simulink model "fboard_xaui"  (Simulink 6.2)
settings: Solver=FixedStepDiscrete  SolverMode=SingleTasking  StartTime=0.0  StopTime=10.0  FixedStep=1  RelTol=1e-3
libraries: xbsIndex_r3 x338, fb_xaui x1, newfft_library x1
(part 1 of 3)
settings Model: LastModifiedBy=mdexter
settings DebuggingCC: SolverPrmCheckMsg=warning

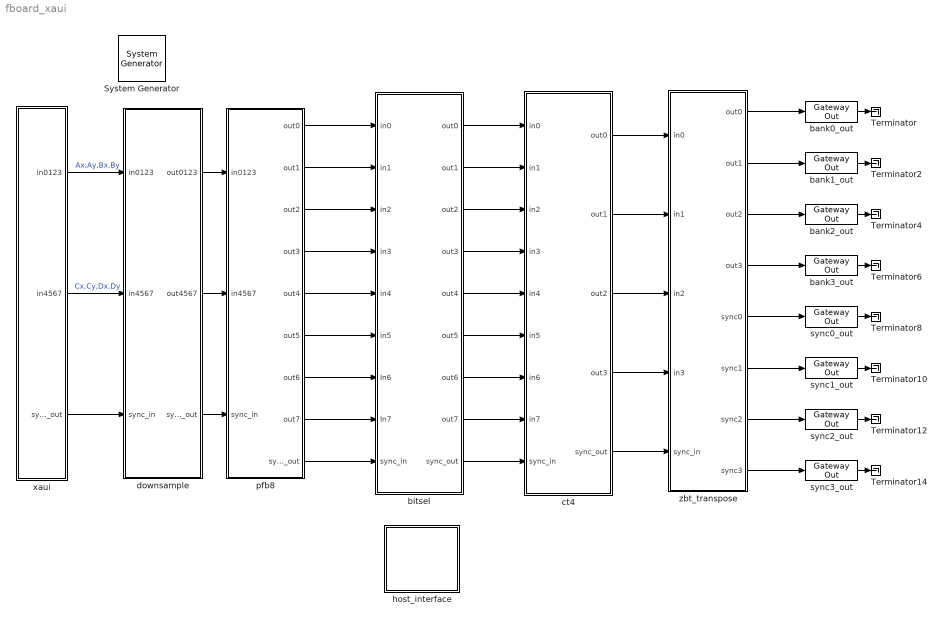
== system fboard_xaui ==
  " System Generator" : xbsIndex_r3/ System Generator  Tag=genX  xilinxfamily=Virtex2P  part=xc2vp40  speed=-6  package=ff1152  synthesis_tool=XST  directory=./netlist  testbench=off  simulink_period=1  sysclk_period=100  incr_netlist=off  trim_vbits=Everywhere in SubSystem  dbl_ovrd=According to Block Masks  core_generation=According to Block Masks  run_coregen=off  deprecated_control=off  eval_field=0
      settings: AttributesFormatString=System\nGenerator
  Terminator{,2,4,6,8,10,12,14} (8 alike) : Terminator
  bank0_out : xbsIndex_r3/Gateway Out  output_type=Double  nbits=8  bin_pt=6  arith_type=Boolean  quantization=Truncate  overflow=Wrap  hdl_port=on  timing_constraint=None  locs_specified=off  LOCs={}  needs_fixed_name=off  show_param=off
      settings: xl_area=[0, 0, 0, 0, 0, 0, 0]
  bank1_out : xbsIndex_r3/Gateway Out  output_type=Double  nbits=8  bin_pt=6  arith_type=Boolean  quantization=Truncate  overflow=Wrap  hdl_port=on  timing_constraint=None  locs_specified=off  LOCs={}  needs_fixed_name=off  show_param=off
      settings: xl_area=[0, 0, 0, 0, 0, 0, 0]
  bank2_out : xbsIndex_r3/Gateway Out  output_type=Double  nbits=8  bin_pt=6  arith_type=Boolean  quantization=Truncate  overflow=Wrap  hdl_port=on  timing_constraint=None  locs_specified=off  LOCs={}  needs_fixed_name=off  show_param=off
      settings: xl_area=[0, 0, 0, 0, 0, 0, 0]
  bank3_out : xbsIndex_r3/Gateway Out  output_type=Double  nbits=8  bin_pt=6  arith_type=Boolean  quantization=Truncate  overflow=Wrap  hdl_port=on  timing_constraint=None  locs_specified=off  LOCs={}  needs_fixed_name=off  show_param=off
      settings: xl_area=[0, 0, 0, 0, 0, 0, 0]
  bitsel : Subsystem
  ct4 : Subsystem
  downsample : Subsystem
  host_interface : Subsystem
  pfb8 : Subsystem
  sync0_out : xbsIndex_r3/Gateway Out  output_type=Double  nbits=8  bin_pt=6  arith_type=Boolean  quantization=Truncate  overflow=Wrap  hdl_port=on  timing_constraint=None  locs_specified=off  LOCs={}  needs_fixed_name=off  show_param=off
      settings: xl_area=[0, 0, 0, 0, 0, 0, 0]
  sync1_out : xbsIndex_r3/Gateway Out  output_type=Double  nbits=8  bin_pt=6  arith_type=Boolean  quantization=Truncate  overflow=Wrap  hdl_port=on  timing_constraint=None  locs_specified=off  LOCs={}  needs_fixed_name=off  show_param=off
      settings: xl_area=[0, 0, 0, 0, 0, 0, 0]
  sync2_out : xbsIndex_r3/Gateway Out  output_type=Double  nbits=8  bin_pt=6  arith_type=Boolean  quantization=Truncate  overflow=Wrap  hdl_port=on  timing_constraint=None  locs_specified=off  LOCs={}  needs_fixed_name=off  show_param=off
      settings: xl_area=[0, 0, 0, 0, 0, 0, 0]
  sync3_out : xbsIndex_r3/Gateway Out  output_type=Double  nbits=8  bin_pt=6  arith_type=Boolean  quantization=Truncate  overflow=Wrap  hdl_port=on  timing_constraint=None  locs_specified=off  LOCs={}  needs_fixed_name=off  show_param=off
      settings: xl_area=[0, 0, 0, 0, 0, 0, 0]
  xaui : Subsystem
  zbt_transpose : Subsystem
  wires:
  pfb8/1(out0) -> bitsel/1(in0)
  pfb8/2(out1) -> bitsel/2(in1)
  pfb8/3(out2) -> bitsel/3(in2)
  pfb8/4(out3) -> bitsel/4(in3)
  pfb8/5(out4) -> bitsel/5(in4)
  pfb8/6(out5) -> bitsel/6(in5)
  pfb8/7(out6) -> bitsel/7(In6)
  pfb8/8(out7) -> bitsel/8(In7)
  pfb8/9(sync_out) -> bitsel/9(sync_in)
  bitsel/1(out0) -> ct4/1(in0)
  ct4/1(out0) -> zbt_transpose/1("in0\t")
  ct4/2(out1) -> zbt_transpose/2(in1)
  ct4/3(out2) -> zbt_transpose/3(in2)
  ct4/4(out3) -> zbt_transpose/4(in3)
  ct4/5(sync_out) -> zbt_transpose/5(sync_in)
  zbt_transpose/1(out0) -> bank0_out/1
  zbt_transpose/2(out1) -> bank1_out/1
  zbt_transpose/3(out2) -> bank2_out/1
  zbt_transpose/4(out3) -> bank3_out/1
  zbt_transpose/5(sync0) -> sync0_out/1
  zbt_transpose/6(sync1) -> sync1_out/1
  zbt_transpose/7(sync2) -> sync2_out/1
  zbt_transpose/8(sync3) -> sync3_out/1
  bitsel/2(out1) -> ct4/2(in1)
  bitsel/3(out2) -> ct4/3(in2)
  bitsel/4(out3) -> ct4/4(in3)
  bitsel/5(out4) -> ct4/5(in4)
  bitsel/6(out5) -> ct4/6(in5)
  bitsel/7(out6) -> ct4/7(in6)
  bitsel/8(out7) -> ct4/8(in7)
  bitsel/9(sync_out) -> ct4/9(sync_in)
  bank0_out/1 -> Terminator/1
  bank1_out/1 -> Terminator2/1
  bank2_out/1 -> Terminator4/1
  bank3_out/1 -> Terminator6/1
  sync0_out/1 -> Terminator8/1
  sync1_out/1 -> Terminator10/1
  sync2_out/1 -> Terminator12/1
  sync3_out/1 -> Terminator14/1
  xaui/1(in0123) -> downsample/1(in0123)  "Ax,Ay,Bx,By"
  xaui/2(in4567) -> downsample/2(in4567)  "Cx,Cy,Dx,Dy"
  xaui/3(sync_out) -> downsample/3(sync_in)
  downsample/1(out0123) -> pfb8/1(in0123)
  downsample/2(out4567) -> pfb8/2(in4567)
  downsample/3(sync_out) -> pfb8/3(sync_in)

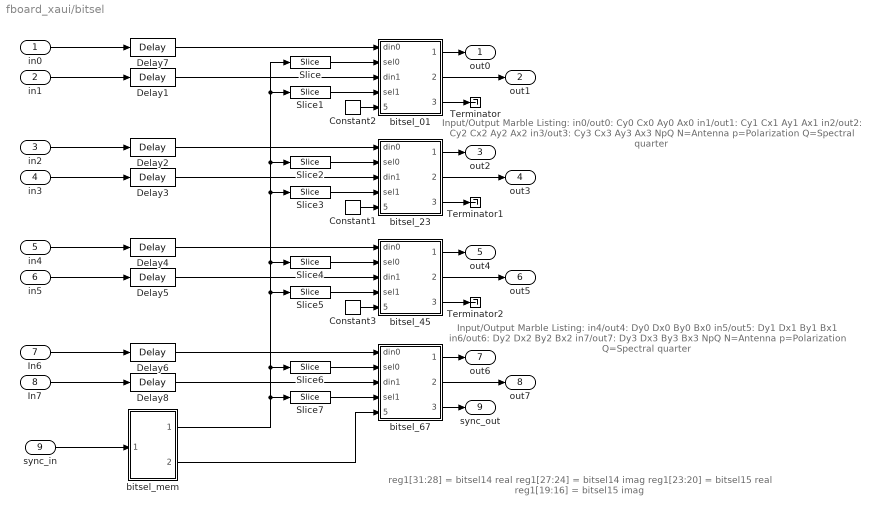
== system fboard_xaui/bitsel ==
  note: Input/Output Marble Listing:
      |
      | in0/out0: Cy0 Cx0 Ay0 Ax0
      | in1/out1: Cy1 Cx1 Ay1 Ax1
      | in2/out2: Cy2 Cx2 Ay2 Ax2
      | in3/out3: Cy3 Cx3 Ay3 Ax3
      |
      | NpQ
      | N=Antenna
      | p=Polarization
      | Q=Spectral quarter
  note: Input/Output Marble Listing:
      |
      | in4/out4: Dy0 Dx0 By0 Bx0
      | in5/out5: Dy1 Dx1 By1 Bx1
      | in6/out6: Dy2 Dx2 By2 Bx2
      | in7/out7: Dy3 Dx3 By3 Bx3
      |
      | NpQ
      | N=Antenna
      | p=Polarization
      | Q=Spectral quarter
  note: reg1[31:28] = bitsel14 real
      | reg1[27:24] = bitsel14 imag
      | reg1[23:20] = bitsel15 real
      | reg1[19:16] = bitsel15 imag
  in0 : Inport  Port=1  LatchInput=off
  in1 : Inport  Port=2  LatchInput=off
  in2 : Inport  Port=3  LatchInput=off
  in3 : Inport  Port=4  LatchInput=off
  in4 : Inport  Port=5  LatchInput=off
  in5 : Inport  Port=6  LatchInput=off
  In6 : Inport  Port=7  LatchInput=off
  In7 : Inport  Port=8  LatchInput=off
  sync_in : Inport  Port=9  LatchInput=off
  Constant1 : xbsIndex_r3/Constant  const=0  equ=P=C  arith_type=Boolean  n_bits=1  bin_pt=0  opselect=C  inp2=PCIN>>17  opr=+  inp1=P  carry=CIN  iostate=0  explicit_period=on  period=1  dbl_ovrd=off
  Constant2 : xbsIndex_r3/Constant  const=0  equ=P=C  arith_type=Boolean  n_bits=1  bin_pt=0  opselect=C  inp2=PCIN>>17  opr=+  inp1=P  carry=CIN  iostate=0  explicit_period=on  period=1  dbl_ovrd=off
  Constant3 : xbsIndex_r3/Constant  const=0  equ=P=C  arith_type=Boolean  n_bits=1  bin_pt=0  opselect=C  inp2=PCIN>>17  opr=+  inp1=P  carry=CIN  iostate=0  explicit_period=on  period=1  dbl_ovrd=off
  Delay{1..8} (8 alike) : xbsIndex_r3/Delay  latency=4  reg_retiming=off  explicit_period=off  period=1  en=off  accept_only_valid=off  init_zero=on  dbl_ovrd=off  show_param=off
      settings: xl_area=[0, 0, 0, 0, 0, 0, 0]
  Slice : xbsIndex_r3/Slice  mode=Lower Bit Location + Width  nbits=4  bit1=0  base1=MSB of Input  bit0=0  base0=LSB of Input  boolean_output=off  explicit_period=off  period=1  dbl_ovrd=off
  Slice1 : xbsIndex_r3/Slice  mode=Lower Bit Location + Width  nbits=4  bit1=0  base1=MSB of Input  bit0=4  base0=LSB of Input  boolean_output=off  explicit_period=off  period=1  dbl_ovrd=off
  Slice2 : xbsIndex_r3/Slice  mode=Lower Bit Location + Width  nbits=4  bit1=0  base1=MSB of Input  bit0=8  base0=LSB of Input  boolean_output=off  explicit_period=off  period=1  dbl_ovrd=off
  Slice3 : xbsIndex_r3/Slice  mode=Lower Bit Location + Width  nbits=4  bit1=0  base1=MSB of Input  bit0=12  base0=LSB of Input  boolean_output=off  explicit_period=off  period=1  dbl_ovrd=off
  Slice4 : xbsIndex_r3/Slice  mode=Lower Bit Location + Width  nbits=4  bit1=0  base1=MSB of Input  bit0=16  base0=LSB of Input  boolean_output=off  explicit_period=off  period=1  dbl_ovrd=off
  Slice5 : xbsIndex_r3/Slice  mode=Lower Bit Location + Width  nbits=4  bit1=0  base1=MSB of Input  bit0=20  base0=LSB of Input  boolean_output=off  explicit_period=off  period=1  dbl_ovrd=off
  Slice6 : xbsIndex_r3/Slice  mode=Lower Bit Location + Width  nbits=4  bit1=0  base1=MSB of Input  bit0=24  base0=LSB of Input  boolean_output=off  explicit_period=off  period=1  dbl_ovrd=off
  Slice7 : xbsIndex_r3/Slice  mode=Lower Bit Location + Width  nbits=4  bit1=0  base1=MSB of Input  bit0=28  base0=LSB of Input  boolean_output=off  explicit_period=off  period=1  dbl_ovrd=off
  Terminator : Terminator
  Terminator1 : Terminator
  Terminator2 : Terminator
  bitsel_01 : Subsystem
  bitsel_23 : Subsystem
  bitsel_45 : Subsystem
  bitsel_67 : Subsystem
  bitsel_mem : Subsystem
      settings: AttributesFormatString=Latency=4
  out0 : Outport
  out1 : Outport  Port=2
  out2 : Outport  Port=3
  out3 : Outport  Port=4
  out4 : Outport  Port=5
  out5 : Outport  Port=6
  out6 : Outport  Port=7
  out7 : Outport  Port=8
  sync_out : Outport  Port=9
  wires:
  in0/1 -> Delay7/1
  bitsel_01/1(dout0) -> out0/1
  in1/1 -> Delay1/1
  in2/1 -> Delay2/1
  in3/1 -> Delay3/1
  in4/1 -> Delay4/1
  in5/1 -> Delay5/1
  In6/1 -> Delay6/1
  In7/1 -> Delay8/1
  bitsel_mem/2(sync_out) -> bitsel_67/5(sync_in)
  Slice/1 -> bitsel_01/2(sel0)
  Slice1/1 -> bitsel_01/4(sel1)
  Slice2/1 -> bitsel_23/2(sel0)
  Slice3/1 -> bitsel_23/4(sel1)
  Slice4/1 -> bitsel_45/2(sel0)
  Slice5/1 -> bitsel_45/4(sel1)
  Slice6/1 -> bitsel_67/2(sel0)
  Slice7/1 -> bitsel_67/4(sel1)
  bitsel_mem/1(bitsel) -> Slice5/1, Slice4/1, Slice3/1, Slice2/1, Slice/1, Slice1/1, Slice6/1, Slice7/1
  bitsel_01/3(sync_out) -> Terminator/1
  bitsel_01/2(dout1) -> out1/1
  bitsel_23/1(dout0) -> out2/1
  bitsel_23/3(sync_out) -> Terminator1/1
  bitsel_23/2(dout1) -> out3/1
  bitsel_45/1(dout0) -> out4/1
  bitsel_45/3(sync_out) -> Terminator2/1
  bitsel_45/2(dout1) -> out5/1
  bitsel_67/1(dout0) -> out6/1
  bitsel_67/2(dout1) -> out7/1
  bitsel_67/3(sync_out) -> sync_out/1
  sync_in/1 -> bitsel_mem/1(sync_in)
  Constant2/1 -> bitsel_01/5(sync_in)
  Constant3/1 -> bitsel_45/5(sync_in)
  Constant1/1 -> bitsel_23/5(sync_in)
  Delay7/1 -> bitsel_01/1(din0)
  Delay1/1 -> bitsel_01/3(din1)
  Delay2/1 -> bitsel_23/1(din0)
  Delay3/1 -> bitsel_23/3(din1)
  Delay4/1 -> bitsel_45/1(din0)
  Delay5/1 -> bitsel_45/3(din1)
  Delay6/1 -> bitsel_67/1(din0)
  Delay8/1 -> bitsel_67/3(din1)

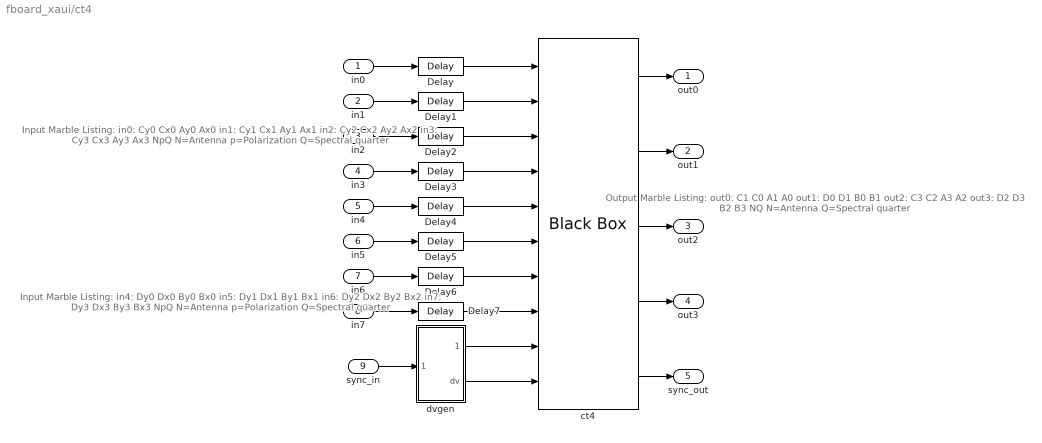
== system fboard_xaui/ct4 ==
  note: Input Marble Listing:
      |
      | in0: Cy0 Cx0 Ay0 Ax0
      | in1: Cy1 Cx1 Ay1 Ax1
      | in2: Cy2 Cx2 Ay2 Ax2
      | in3: Cy3 Cx3 Ay3 Ax3
      |
      | NpQ
      | N=Antenna
      | p=Polarization
      | Q=Spectral quarter
  note: Input Marble Listing:
      |
      | in4: Dy0 Dx0 By0 Bx0
      | in5: Dy1 Dx1 By1 Bx1
      | in6: Dy2 Dx2 By2 Bx2
      | in7: Dy3 Dx3 By3 Bx3
      |
      | NpQ
      | N=Antenna
      | p=Polarization
      | Q=Spectral quarter
  note: Output Marble Listing:
      |
      | out0: C1 C0 A1 A0
      | out1: D0 D1 B0 B1
      | out2: C3 C2 A3 A2
      | out3: D2 D3 B2 B3
      |
      | NQ
      | N=Antenna
      | Q=Spectral quarter
  in0 : Inport  Port=1  LatchInput=off
  in1 : Inport  Port=2  LatchInput=off
  in2 : Inport  Port=3  LatchInput=off
  in3 : Inport  Port=4  LatchInput=off
  in4 : Inport  Port=5  LatchInput=off
  in5 : Inport  Port=6  LatchInput=off
  in6 : Inport  Port=7  LatchInput=off
  in7 : Inport  Port=8  LatchInput=off
  sync_in : Inport  Port=9  LatchInput=off
  Delay{,1..7} (8 alike) : xbsIndex_r3/Delay  latency=3  reg_retiming=off  explicit_period=off  period=1  en=off  accept_only_valid=off  init_zero=on  dbl_ovrd=off  show_param=off
      settings: xl_area=[0, 0, 0, 0, 0, 0, 0]
  ct4 : xbsIndex_r3/Black Box  init_code=ct4_dv_config  sim_method=Inactive  show_param=off
      settings: xl_area=[0, 0, 0, 0, 0, 0, 0]
  dvgen : Subsystem
      settings: AttributesFormatString=Latency=3
  out0 : Outport
  out1 : Outport  Port=2
  out2 : Outport  Port=3
  out3 : Outport  Port=4
  sync_out : Outport  Port=5
  wires:
  in0/1 -> Delay/1
  ct4/1 -> out0/1
  in1/1 -> Delay1/1
  ct4/2 -> out1/1
  in2/1 -> Delay2/1
  ct4/3 -> out2/1
  in3/1 -> Delay3/1
  ct4/4 -> out3/1
  in4/1 -> Delay4/1
  ct4/5 -> sync_out/1
  in5/1 -> Delay5/1
  in6/1 -> Delay6/1
  in7/1 -> Delay7/1
  dvgen/1(sync_out) -> ct4/9
  dvgen/2(dv) -> ct4/10
  sync_in/1 -> dvgen/1(sync_in)
  Delay/1 -> ct4/1
  Delay1/1 -> ct4/2
  Delay2/1 -> ct4/3
  Delay3/1 -> ct4/4
  Delay4/1 -> ct4/5
  Delay5/1 -> ct4/6
  Delay6/1 -> ct4/7
  Delay7/1 -> ct4/8

== system fboard_xaui/downsample ==
  note: The down-sampling step down-samples the sync pulse to the
      | slower rate and down-samples data to the slower rate as well.
  note: sync_in (1/1 rate): _S_____________
      | data_in (1/1 rate): YZ0123456789ABC
      | sync_out (1/2 rate): _____SS________
      | data_out (1/2 rate): TVVXXZZ11335577
      | dv (1/2 rate): 010101010101010
  in0123 : Inport  Port=1  LatchInput=off
  in4567 : Inport  Port=2  LatchInput=off
  sync_in : Inport  Port=3  LatchInput=off
  Delay1 : xbsIndex_r3/Delay  latency=3  reg_retiming=off  explicit_period=off  period=1  en=off  accept_only_valid=off  init_zero=on  dbl_ovrd=off  show_param=off
      settings: xl_area=[0, 0, 0, 0, 0, 0, 0]
  Delay2 : xbsIndex_r3/Delay  latency=3  reg_retiming=off  explicit_period=off  period=1  en=off  accept_only_valid=off  init_zero=on  dbl_ovrd=off  show_param=off
      settings: xl_area=[0, 0, 0, 0, 0, 0, 0]
  Register : xbsIndex_r3/Register  init=0  reg_only_valid=off  explicit_period=off  period=1  rst=off  en=on  out_en=off  dbl_ovrd=off  show_param=off
      settings: xl_area=[0, 0, 0, 0, 0, 0, 0]
  Register1 : xbsIndex_r3/Register  init=0  reg_only_valid=off  explicit_period=off  period=1  rst=off  en=on  out_en=off  dbl_ovrd=off  show_param=off
      settings: xl_area=[0, 0, 0, 0, 0, 0, 0]
  Register2 : xbsIndex_r3/Register  init=0  reg_only_valid=off  explicit_period=off  period=1  rst=off  en=on  out_en=off  dbl_ovrd=off  show_param=off
      settings: xl_area=[0, 0, 0, 0, 0, 0, 0]
  dvgen : Subsystem
      settings: AttributesFormatString=Latency=3
  out0123 : Outport
  out4567 : Outport  Port=2
  sync_out : Outport  Port=3
  wires:
  in0123/1 -> Delay1/1
  in4567/1 -> Delay2/1
  sync_in/1 -> dvgen/1(sync_in)
  Register/1 -> out0123/1
  Register1/1 -> out4567/1
  Register2/1 -> sync_out/1
  dvgen/1(sync_out) -> Register2/1
  dvgen/2(dv) -> Register2/2, Register/2, Register1/2
  Delay1/1 -> Register/1
  Delay2/1 -> Register1/1

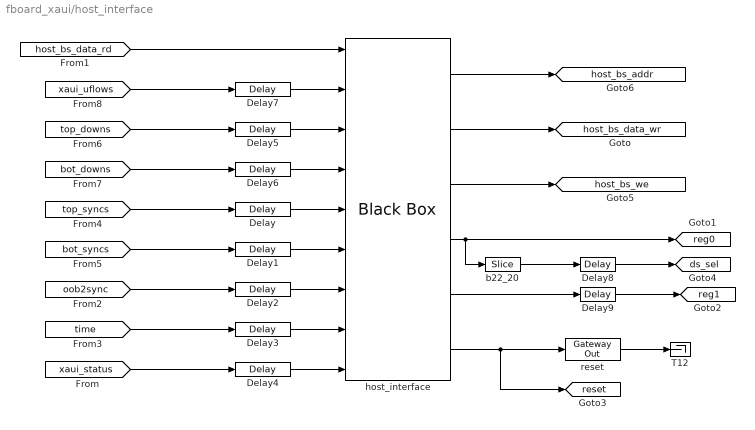
== system fboard_xaui/host_interface ==
  Delay{,1..7} (8 alike) : xbsIndex_r3/Delay  latency=1  reg_retiming=off  explicit_period=off  period=1  en=off  accept_only_valid=off  init_zero=on  dbl_ovrd=off  show_param=off
      settings: xl_area=[0, 0, 0, 0, 0, 0, 0]
  Delay8 : xbsIndex_r3/Delay  latency=3  reg_retiming=on  explicit_period=off  period=1  en=off  accept_only_valid=off  init_zero=on  dbl_ovrd=off  show_param=off
      settings: xl_area=[0, 0, 0, 0, 0, 0, 0]
  Delay9 : xbsIndex_r3/Delay  latency=3  reg_retiming=on  explicit_period=off  period=1  en=off  accept_only_valid=off  init_zero=on  dbl_ovrd=off  show_param=off
      settings: xl_area=[0, 0, 0, 0, 0, 0, 0]
  T12 : Terminator
  b22_20 : xbsIndex_r3/Slice  mode=Lower Bit Location + Width  nbits=3  bit1=0  base1=MSB of Input  bit0=20  base0=LSB of Input  boolean_output=off  explicit_period=off  period=1  dbl_ovrd=off
  host_interface : xbsIndex_r3/Black Box  init_code=host_interface_config  sim_method=Inactive  show_param=off
      settings: xl_area=[0, 0, 0, 0, 0, 0, 0]
  reset : xbsIndex_r3/Gateway Out  output_type=Double  nbits=8  bin_pt=6  arith_type=Boolean  quantization=Truncate  overflow=Wrap  hdl_port=on  timing_constraint=None  locs_specified=off  LOCs={}  needs_fixed_name=off  show_param=off
      settings: xl_area=[0, 0, 0, 0, 0, 0, 0]
  tag scope: ds_sel=global, host_bs_addr=global, host_bs_data_wr=global, host_bs_we=global, reg0=global, reg1=global, reset=global
  wires:
  reset/1 -> T12/1
  [host_bs_data_rd] -> host_interface/1
  host_interface/6 -> reset/1, [reset]
  host_interface/2 -> [host_bs_data_wr]
  [top_syncs] -> Delay/1
  [bot_syncs] -> Delay1/1
  [oob2sync] -> Delay2/1
  [time] -> Delay3/1
  [xaui_status] -> Delay4/1
  [top_downs] -> Delay5/1
  [bot_downs] -> Delay6/1
  host_interface/4 -> [reg0], b22_20/1
  host_interface/5 -> Delay9/1
  [xaui_uflows] -> Delay7/1
  Delay7/1 -> host_interface/2
  Delay5/1 -> host_interface/3
  Delay6/1 -> host_interface/4
  Delay/1 -> host_interface/5
  Delay1/1 -> host_interface/6
  Delay2/1 -> host_interface/7
  Delay3/1 -> host_interface/8
  Delay4/1 -> host_interface/9
  b22_20/1 -> Delay8/1
  host_interface/3 -> [host_bs_we]
  host_interface/1 -> [host_bs_addr]
  Delay8/1 -> [ds_sel]
  Delay9/1 -> [reg1]

== system fboard_xaui/pfb8 ==
  in0123 : Inport  Port=1  LatchInput=off
  in4567 : Inport  Port=2  LatchInput=off
  sync_in : Inport  Port=3  LatchInput=off
  b64x1_b16x4_bot : Subsystem
  b64x1_b16x4_top : Subsystem
  fir8 : Subsystem  mask{fb_ntaps=4}
      mask prompts: fb_ntaps "Number of taps"
  pfb_fft8 : Subsystem
  out0 : Outport
  out1 : Outport  Port=2
  out2 : Outport  Port=3
  out3 : Outport  Port=4
  out4 : Outport  Port=5
  out5 : Outport  Port=6
  out6 : Outport  Port=7
  out7 : Outport  Port=8
  sync_out : Outport  Port=9
  wires:
  fir8/8(out7) -> pfb_fft8/8(in7)
  fir8/7(out6) -> pfb_fft8/7(in6)
  fir8/9(sync_out) -> pfb_fft8/9(sync_in)
  fir8/6(out5) -> pfb_fft8/6(in5)
  fir8/5(out4) -> pfb_fft8/5(in4)
  fir8/4(out3) -> pfb_fft8/4(in3)
  fir8/3(out2) -> pfb_fft8/3(in2)
  fir8/2(out1) -> pfb_fft8/2(in1)
  fir8/1(out0) -> pfb_fft8/1(in0)
  b64x1_b16x4_top/2(dout1) -> fir8/2(in1)
  b64x1_b16x4_top/1(dout0) -> fir8/1(in0)
  b64x1_b16x4_bot/4(dout3) -> fir8/8(in7)
  b64x1_b16x4_bot/3(dout2) -> fir8/7(in6)
  b64x1_b16x4_bot/2(dout1) -> fir8/6(in5)
  b64x1_b16x4_bot/1(dout0) -> fir8/5(in4)
  b64x1_b16x4_top/4(dout3) -> fir8/4(in3)
  b64x1_b16x4_top/3(dout2) -> fir8/3(in2)
  pfb_fft8/1(out0) -> out0/1
  pfb_fft8/2(out1) -> out1/1
  in0123/1 -> b64x1_b16x4_top/1(din)
  pfb_fft8/3(out2) -> out2/1
  pfb_fft8/4(out3) -> out3/1
  pfb_fft8/5(out4) -> out4/1
  pfb_fft8/6(out5) -> out5/1
  in4567/1 -> b64x1_b16x4_bot/1(din)
  pfb_fft8/7(out6) -> out6/1
  pfb_fft8/8(out7) -> out7/1
  pfb_fft8/9(sync_out) -> sync_out/1
  sync_in/1 -> fir8/9(sync_in)

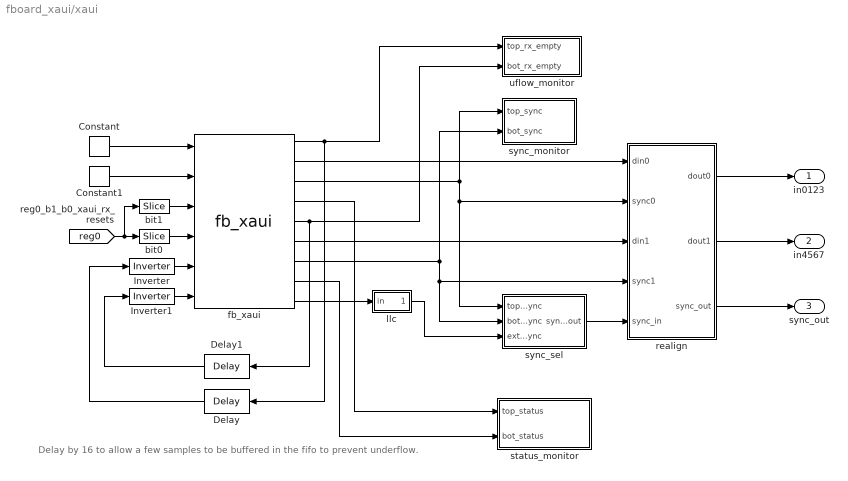
== system fboard_xaui/xaui ==
  note: Delay by 16 to allow a few samples to be
      | buffered in the fifo to prevent underflow.
  Constant : xbsIndex_r3/Constant  const=0  equ=P=C  arith_type=Boolean  n_bits=1  bin_pt=0  opselect=C  inp2=PCIN>>17  opr=+  inp1=P  carry=CIN  iostate=0  explicit_period=on  period=1  dbl_ovrd=off
  Constant1 : xbsIndex_r3/Constant  const=1  equ=P=C  arith_type=Boolean  n_bits=1  bin_pt=0  opselect=C  inp2=PCIN>>17  opr=+  inp1=P  carry=CIN  iostate=0  explicit_period=on  period=1  dbl_ovrd=off
  Delay : xbsIndex_r3/Delay  Orientation=left  latency=16  reg_retiming=off  explicit_period=off  period=1  en=off  accept_only_valid=off  init_zero=on  dbl_ovrd=off  show_param=off
      settings: xl_area=[0, 0, 0, 0, 0, 0, 0]
  Delay1 : xbsIndex_r3/Delay  Orientation=left  latency=16  reg_retiming=off  explicit_period=off  period=1  en=off  accept_only_valid=off  init_zero=on  dbl_ovrd=off  show_param=off
      settings: xl_area=[0, 0, 0, 0, 0, 0, 0]
  Inverter : xbsIndex_r3/Inverter  latency=0  explicit_period=off  period=1  en=off  dbl_ovrd=off  show_param=off
      settings: xl_area=[0, 0, 0, 0, 0, 0, 0]
  Inverter1 : xbsIndex_r3/Inverter  latency=0  explicit_period=off  period=1  en=off  dbl_ovrd=off  show_param=off
      settings: xl_area=[0, 0, 0, 0, 0, 0, 0]
  bit0 : xbsIndex_r3/Slice  mode=Lower Bit Location + Width  nbits=1  bit1=12  base1=MSB of Input  bit0=0  base0=LSB of Input  boolean_output=on  explicit_period=off  period=1  dbl_ovrd=off
  bit1 : xbsIndex_r3/Slice  mode=Lower Bit Location + Width  nbits=1  bit1=12  base1=MSB of Input  bit0=1  base0=LSB of Input  boolean_output=on  explicit_period=off  period=1  dbl_ovrd=off
  fb_xaui : fb_xaui/fb_xaui
  llc : Subsystem
  realign : Subsystem
  status_monitor : Subsystem
  sync_monitor : Subsystem
  sync_sel : Subsystem
  uflow_monitor : Subsystem
  in0123 : Outport
  in4567 : Outport  Port=2
  sync_out : Outport  Port=3
  wires:
  Constant/1 -> fb_xaui/1
  Constant1/1 -> fb_xaui/2
  fb_xaui/8 -> status_monitor/2(bot_status)
  fb_xaui/4 -> status_monitor/1(top_status)
  fb_xaui/2 -> realign/1(din0)
  fb_xaui/3 -> sync_monitor/1(top_sync), sync_sel/1(top_sync), realign/2(sync0)
  fb_xaui/6 -> realign/3(din1)
  fb_xaui/7 -> sync_monitor/2(bot_sync), realign/4(sync1), sync_sel/2(bot_sync)
  realign/1(dout0) -> in0123/1
  realign/2(dout1) -> in4567/1
  realign/3(sync_out) -> sync_out/1
  sync_sel/1(sync_out) -> realign/5(sync_in)
  fb_xaui/1 -> uflow_monitor/1(top_rx_empty), Delay/1
  fb_xaui/5 -> uflow_monitor/2(bot_rx_empty), Delay1/1
  [reg0] -> bit0/1, bit1/1
  bit1/1 -> fb_xaui/3
  bit0/1 -> fb_xaui/4
  Delay/1 -> Inverter/1
  Delay1/1 -> Inverter1/1
  Inverter/1 -> fb_xaui/5
  Inverter1/1 -> fb_xaui/6
  fb_xaui/9 -> llc/1(in)
  llc/1(out) -> sync_sel/3(ext_sync)

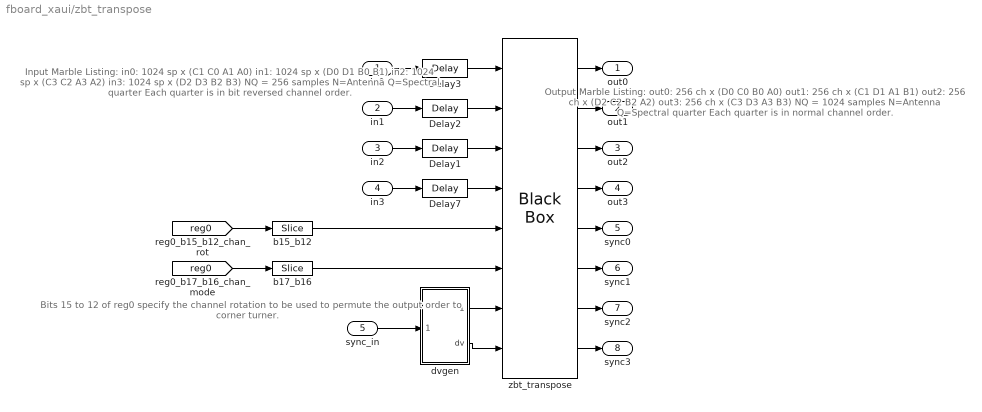
== system fboard_xaui/zbt_transpose ==
  note: Input Marble Listing:
      |
      | in0: 1024 sp x (C1 C0 A1 A0)
      | in1: 1024 sp x (D0 D1 B0 B1)
      | in2: 1024 sp x (C3 C2 A3 A2)
      | in3: 1024 sp x (D2 D3 B2 B3)
      |
      | NQ = 256 samples
      |
      | N=Antenna
      | Q=Spectral quarter
      |
      | Each quarter is in bit
      | reversed channel order.
  note: Output Marble Listing:
      |
      | out0: 256 ch x (D0 C0 B0 A0)
      | out1: 256 ch x (C1 D1 A1 B1)
      | out2: 256 ch x (D2 C2 B2 A2)
      | out3: 256 ch x (C3 D3 A3 B3)
      |
      | NQ = 1024 samples
      |
      | N=Antenna
      | Q=Spectral quarter
      |
      | Each quarter is in
      | normal channel order.
  note: Bits 15 to 12 of reg0
      | specify the channel rotation
      | to be used to permute the
      | output order to corner turner.
  "in0\t" : Inport  Port=1  LatchInput=off
  in1 : Inport  Port=2  LatchInput=off
  in2 : Inport  Port=3  LatchInput=off
  in3 : Inport  Port=4  LatchInput=off
  sync_in : Inport  Port=5  LatchInput=off
  Delay{1..3,7} (4 alike) : xbsIndex_r3/Delay  latency=3  reg_retiming=off  explicit_period=off  period=1  en=off  accept_only_valid=off  init_zero=on  dbl_ovrd=off  show_param=off
      settings: xl_area=[0, 0, 0, 0, 0, 0, 0]
  b15_b12 : xbsIndex_r3/Slice  mode=Lower Bit Location + Width  nbits=4  bit1=12  base1=MSB of Input  bit0=12  base0=LSB of Input  boolean_output=off  explicit_period=off  period=1  dbl_ovrd=off
  b17_b16 : xbsIndex_r3/Slice  mode=Lower Bit Location + Width  nbits=2  bit1=12  base1=MSB of Input  bit0=16  base0=LSB of Input  boolean_output=off  explicit_period=off  period=1  dbl_ovrd=off
  dvgen : Subsystem
      settings: AttributesFormatString=Latency=3
  zbt_transpose : xbsIndex_r3/Black Box  init_code=zbt_transpose_config  sim_method=Inactive  show_param=off
      settings: xl_area=[0, 0, 0, 0, 0, 0, 0]
  out0 : Outport
  out1 : Outport  Port=2
  out2 : Outport  Port=3
  out3 : Outport  Port=4
  sync0 : Outport  Port=5
  sync1 : Outport  Port=6
  sync2 : Outport  Port=7
  sync3 : Outport  Port=8
  wires:
  zbt_transpose/1 -> out0/1
  "in0\t"/1 -> Delay3/1
  zbt_transpose/2 -> out1/1
  in1/1 -> Delay2/1
  zbt_transpose/3 -> out2/1
  zbt_transpose/4 -> out3/1
  in2/1 -> Delay1/1
  zbt_transpose/5 -> sync0/1
  in3/1 -> Delay7/1
  zbt_transpose/6 -> sync1/1
  zbt_transpose/7 -> sync2/1
  zbt_transpose/8 -> sync3/1
  [reg0] -> b15_b12/1
  [reg0] -> b17_b16/1
  b15_b12/1 -> zbt_transpose/5
  b17_b16/1 -> zbt_transpose/6
  Delay7/1 -> zbt_transpose/4
  Delay1/1 -> zbt_transpose/3
  Delay2/1 -> zbt_transpose/2
  Delay3/1 -> zbt_transpose/1
  dvgen/1(sync_out) -> zbt_transpose/7
  dvgen/2(dv) -> zbt_transpose/8
  sync_in/1 -> dvgen/1(sync_in)

== system fboard_xaui/bitsel/bitsel_01 ==
  din0 : Inport  Port=1  LatchInput=off
  sel0 : Inport  Port=2  LatchInput=off
  din1 : Inport  Port=3  LatchInput=off
  sel1 : Inport  Port=4  LatchInput=off
  sync_in : Inport  Port=5  LatchInput=off
  Constant : xbsIndex_r3/Constant  const=0  equ=P=C  arith_type=Boolean  n_bits=1  bin_pt=0  opselect=C  inp2=PCIN>>17  opr=+  inp1=P  carry=CIN  iostate=0  explicit_period=on  period=1  dbl_ovrd=off
  Terminator : Terminator
  bitsel_0 : xbsIndex_r3/Black Box  init_code=bitsel_config  sim_method=Inactive  show_param=off
      settings: xl_area=[0, 0, 0, 0, 0, 0, 0]
  bitsel_1 : xbsIndex_r3/Black Box  init_code=bitsel_config  sim_method=Inactive  show_param=off
      settings: xl_area=[0, 0, 0, 0, 0, 0, 0]
  dout0 : Outport
  dout1 : Outport  Port=2
  sync_out : Outport  Port=3
  wires:
  din0/1 -> bitsel_0/1
  din1/1 -> bitsel_1/1
  sel0/1 -> bitsel_0/2
  bitsel_0/1 -> dout0/1
  sel1/1 -> bitsel_1/2
  bitsel_1/1 -> dout1/1
  sync_in/1 -> bitsel_1/4
  bitsel_1/2 -> sync_out/1
  bitsel_0/2 -> Terminator/1
  Constant/1 -> bitsel_0/4
  [bs1415] -> bitsel_0/3
  [bs1415] -> bitsel_1/3

== system fboard_xaui/bitsel/bitsel_23 ==
  din0 : Inport  Port=1  LatchInput=off
  sel0 : Inport  Port=2  LatchInput=off
  din1 : Inport  Port=3  LatchInput=off
  sel1 : Inport  Port=4  LatchInput=off
  sync_in : Inport  Port=5  LatchInput=off
  Constant : xbsIndex_r3/Constant  const=0  equ=P=C  arith_type=Boolean  n_bits=1  bin_pt=0  opselect=C  inp2=PCIN>>17  opr=+  inp1=P  carry=CIN  iostate=0  explicit_period=on  period=1  dbl_ovrd=off
  Terminator : Terminator
  bitsel_0 : xbsIndex_r3/Black Box  init_code=bitsel_config  sim_method=Inactive  show_param=off
      settings: xl_area=[0, 0, 0, 0, 0, 0, 0]
  bitsel_1 : xbsIndex_r3/Black Box  init_code=bitsel_config  sim_method=Inactive  show_param=off
      settings: xl_area=[0, 0, 0, 0, 0, 0, 0]
  dout0 : Outport
  dout1 : Outport  Port=2
  sync_out : Outport  Port=3
  wires:
  din0/1 -> bitsel_0/1
  din1/1 -> bitsel_1/1
  sel0/1 -> bitsel_0/2
  bitsel_0/1 -> dout0/1
  sel1/1 -> bitsel_1/2
  bitsel_1/1 -> dout1/1
  sync_in/1 -> bitsel_1/4
  bitsel_1/2 -> sync_out/1
  bitsel_0/2 -> Terminator/1
  Constant/1 -> bitsel_0/4
  [bs1415] -> bitsel_0/3
  [bs1415] -> bitsel_1/3

== system fboard_xaui/bitsel/bitsel_45 ==
  din0 : Inport  Port=1  LatchInput=off
  sel0 : Inport  Port=2  LatchInput=off
  din1 : Inport  Port=3  LatchInput=off
  sel1 : Inport  Port=4  LatchInput=off
  sync_in : Inport  Port=5  LatchInput=off
  Constant : xbsIndex_r3/Constant  const=0  equ=P=C  arith_type=Boolean  n_bits=1  bin_pt=0  opselect=C  inp2=PCIN>>17  opr=+  inp1=P  carry=CIN  iostate=0  explicit_period=on  period=1  dbl_ovrd=off
  Terminator : Terminator
  bitsel_0 : xbsIndex_r3/Black Box  init_code=bitsel_config  sim_method=Inactive  show_param=off
      settings: xl_area=[0, 0, 0, 0, 0, 0, 0]
  bitsel_1 : xbsIndex_r3/Black Box  init_code=bitsel_config  sim_method=Inactive  show_param=off
      settings: xl_area=[0, 0, 0, 0, 0, 0, 0]
  dout0 : Outport
  dout1 : Outport  Port=2
  sync_out : Outport  Port=3
  wires:
  din0/1 -> bitsel_0/1
  din1/1 -> bitsel_1/1
  sel0/1 -> bitsel_0/2
  bitsel_0/1 -> dout0/1
  sel1/1 -> bitsel_1/2
  bitsel_1/1 -> dout1/1
  sync_in/1 -> bitsel_1/4
  bitsel_1/2 -> sync_out/1
  bitsel_0/2 -> Terminator/1
  Constant/1 -> bitsel_0/4
  [bs1415] -> bitsel_0/3
  [bs1415] -> bitsel_1/3

== system fboard_xaui/bitsel/bitsel_67 ==
  din0 : Inport  Port=1  LatchInput=off
  sel0 : Inport  Port=2  LatchInput=off
  din1 : Inport  Port=3  LatchInput=off
  sel1 : Inport  Port=4  LatchInput=off
  sync_in : Inport  Port=5  LatchInput=off
  Constant : xbsIndex_r3/Constant  const=0  equ=P=C  arith_type=Boolean  n_bits=1  bin_pt=0  opselect=C  inp2=PCIN>>17  opr=+  inp1=P  carry=CIN  iostate=0  explicit_period=on  period=1  dbl_ovrd=off
  Terminator : Terminator
  bitsel_0 : xbsIndex_r3/Black Box  init_code=bitsel_config  sim_method=Inactive  show_param=off
      settings: xl_area=[0, 0, 0, 0, 0, 0, 0]
  bitsel_1 : xbsIndex_r3/Black Box  init_code=bitsel_config  sim_method=Inactive  show_param=off
      settings: xl_area=[0, 0, 0, 0, 0, 0, 0]
  dout0 : Outport
  dout1 : Outport  Port=2
  sync_out : Outport  Port=3
  wires:
  din0/1 -> bitsel_0/1
  din1/1 -> bitsel_1/1
  sel0/1 -> bitsel_0/2
  bitsel_0/1 -> dout0/1
  sel1/1 -> bitsel_1/2
  bitsel_1/1 -> dout1/1
  sync_in/1 -> bitsel_1/4
  bitsel_1/2 -> sync_out/1
  bitsel_0/2 -> Terminator/1
  Constant/1 -> bitsel_0/4
  [bs1415] -> bitsel_0/3
  [bs1415] -> bitsel_1/3

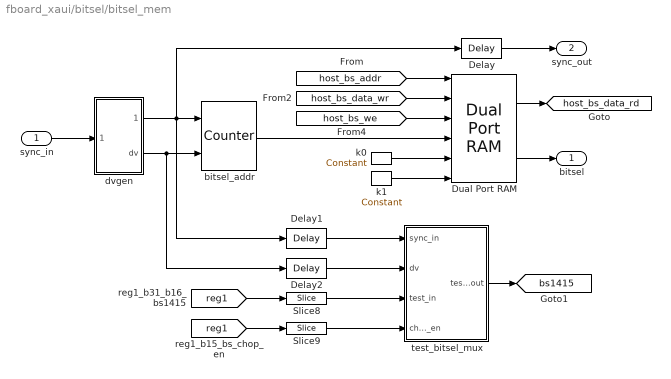
== system fboard_xaui/bitsel/bitsel_mem ==
  sync_in : Inport  Port=1  LatchInput=off
  Delay : xbsIndex_r3/Delay  latency=1  reg_retiming=off  explicit_period=off  period=1  en=off  accept_only_valid=off  init_zero=on  dbl_ovrd=off  show_param=off
      settings: xl_area=[0, 0, 0, 0, 0, 0, 0]
  Delay1 : xbsIndex_r3/Delay  latency=1  reg_retiming=off  explicit_period=off  period=1  en=off  accept_only_valid=off  init_zero=on  dbl_ovrd=off  show_param=off
      settings: xl_area=[0, 0, 0, 0, 0, 0, 0]
  Delay2 : xbsIndex_r3/Delay  latency=1  reg_retiming=off  explicit_period=off  period=1  en=off  accept_only_valid=off  init_zero=on  dbl_ovrd=off  show_param=off
      settings: xl_area=[0, 0, 0, 0, 0, 0, 0]
  Dual Port RAM : xbsIndex_r3/Dual Port RAM  depth=1024  initVector=ones(1,1024)*hex2dec('77777777')  write_mode_A=Read After Write  write_mode_B=Read After Write  latency=1  mem_collision=off  init_zero=on  explicit_period=off  period=1  dbl_ovrd=off  rst_a=off  init_a=0  rst_b=off  init_b=0  show_param=on  distributed_mem=off  use_rpm=off  gen_core=off
      settings: xl_area=[0, 0, 0, 0, 0, 0, 0]
  Slice8 : xbsIndex_r3/Slice  mode=Lower Bit Location + Width  nbits=16  bit1=0  base1=MSB of Input  bit0=16  base0=LSB of Input  boolean_output=off  explicit_period=off  period=1  dbl_ovrd=off
  Slice9 : xbsIndex_r3/Slice  mode=Lower Bit Location + Width  nbits=1  bit1=0  base1=MSB of Input  bit0=15  base0=LSB of Input  boolean_output=off  explicit_period=off  period=1  dbl_ovrd=off
  bitsel_addr : xbsIndex_r3/Counter  cnt_type=Free Running  n_bits=10  bin_pt=0  arith_type=Unsigned  start_count=0  cnt_to=Inf  cnt_by_val=1  operation=Up  explicit_period=off  period=1  load_pin=off  rst=on  en=on  dbl_ovrd=off  show_param=off  use_rpm=on  gen_core=off
      settings: xl_area=[0, 0, 0, 0, 0, 0, 0]
  dvgen : Subsystem
      settings: AttributesFormatString=Latency=3
  k0 : xbsIndex_r3/Constant  const=0  equ=P=C  arith_type=Unsigned  n_bits=32  bin_pt=0  opselect=C  inp2=PCIN>>17  opr=+  inp1=P  carry=CIN  iostate=0  explicit_period=on  period=1  dbl_ovrd=off
  k1 : xbsIndex_r3/Constant  const=0  equ=P=C  arith_type=Boolean  n_bits=32  bin_pt=0  opselect=C  inp2=PCIN>>17  opr=+  inp1=P  carry=CIN  iostate=0  explicit_period=on  period=1  dbl_ovrd=off
  test_bitsel_mux : Subsystem
  bitsel : Outport
  sync_out : Outport  Port=2
  tag scope: bs1415=global, host_bs_data_rd=global
  wires:
  bitsel_addr/1 -> Dual Port RAM/4
  k0/1 -> Dual Port RAM/5
  k1/1 -> Dual Port RAM/6
  [host_bs_we] -> Dual Port RAM/3
  Dual Port RAM/1 -> [host_bs_data_rd]
  [host_bs_addr] -> Dual Port RAM/1
  [host_bs_data_wr] -> Dual Port RAM/2
  dvgen/1(sync_out) -> bitsel_addr/1, Delay/1, Delay1/1
  dvgen/2(dv) -> bitsel_addr/2, Delay2/1
  Dual Port RAM/2 -> bitsel/1
  Delay/1 -> sync_out/1
  sync_in/1 -> dvgen/1(sync_in)
  [reg1] -> Slice8/1
  [reg1] -> Slice9/1
  test_bitsel_mux/1(test_out) -> [bs1415]
  Delay1/1 -> test_bitsel_mux/1(sync_in)
  Delay2/1 -> test_bitsel_mux/2(dv)
  Slice8/1 -> test_bitsel_mux/3(test_in)
  Slice9/1 -> test_bitsel_mux/4(chop_en)

== system fboard_xaui/ct4/dvgen ==
  note: This dvgen block generates a dv signal based on sync_in's rising
      | edge and the value of ds_sel (downsample select), which is taken
      | from a global goto tag.  ds_sel can range from 0 to 7.  The dv
      | signal will be asserted for one cycle every 2^ds_sel cycles starting
      | with the first cycle after sync_out's rising edge.  Note that sync_in
      | may be one or many cycles wide, but it should probably be no
      | wider than 2^ds_sel cycles for typical usage.  sync_out is always
      | one cycle wide (corresponding to the first active cycle of sync_in).
  note: == Example Timing Diagrams ==
      |
      | -------  ds_sel == 0  -------
      | sync_in : .S................
      | sync_out : ....S.............
      | dv : 111111111111111111
      |
      | -------  ds_sel == 1  -------
      | sync_in : .S................
      | sync_out : ....S.............
      | dv : XXXX1.1.1.1.1.1.1.
      |
      | -------  ds_sel == 2  -------
      | sync_in : .SSSS.............
      | sync_out : ....S.............
      | dv : XXXX1...1...1...1.
  note: Only honor new ds_sel value
      | on rising edge of sync_in
  sync_in : Inport  Port=1  LatchInput=off
  Constant2 : xbsIndex_r3/Constant  const=0  equ=P=C  arith_type=Unsigned  n_bits=1  bin_pt=0  opselect=C  inp2=PCIN>>17  opr=+  inp1=P  carry=CIN  iostate=0  explicit_period=on  period=1  dbl_ovrd=off
  Counter : xbsIndex_r3/Counter  cnt_type=Free Running  n_bits=7  bin_pt=0  arith_type=Unsigned  start_count=0  cnt_to=Inf  cnt_by_val=1  operation=Up  explicit_period=off  period=1  load_pin=off  rst=on  en=off  dbl_ovrd=off  show_param=on  use_rpm=on  gen_core=off
      settings: xl_area=[0, 0, 0, 0, 0, 0, 0]
  Delay : xbsIndex_r3/Delay  latency=3  reg_retiming=off  explicit_period=off  period=1  en=off  accept_only_valid=off  init_zero=on  dbl_ovrd=off  show_param=off
      settings: xl_area=[0, 0, 0, 0, 0, 0, 0]
  Mux : xbsIndex_r3/Mux  inputs=8  precision=Full  arith_type="Signed  (2's comp)"  n_bits=8  bin_pt=2  quantization=Truncate  overflow=Wrap  latency=1  explicit_period=off  period=1  en=off  dbl_ovrd=off  show_param=off  mux_type=off  use_rpm=off  gen_core=off
      settings: xl_area=[0, 0, 0, 0, 0, 0, 0]
  Register2 : xbsIndex_r3/Register  init=0  reg_only_valid=off  explicit_period=off  period=1  rst=off  en=on  out_en=off  dbl_ovrd=off  show_param=off
      settings: xl_area=[0, 0, 0, 0, 0, 0, 0]
  Relational : xbsIndex_r3/Relational  mode=a=b  latency=1  explicit_period=off  period=1  en=off  dbl_ovrd=off  show_param=on
      settings: xl_area=[0, 0, 0, 0, 0, 0, 0]
  bit_slicer : Subsystem
  edge_detect : Subsystem  mask(Edge Detector){edge=Rising, polarity=Active High, xin=floor([0.5:0.5:5])*0.08, yin={[-1,-1,1,1,1,1,1,1,1,1],[1,1,-1,-1,-1,-1,-1,-1,-1,-1],[-1,-1,1,1,1,1,-1,-1,-1,-1]}, xout=1-floor([5:-0.5:0.5])*0.08, yout={[-1,-1,1,1,-1,-1,-1,-1,-1,-1],[-1,-1,1,1,-1,-1,-1,-1,-1,-1],[-1,-1,1,1,-1,-1,1,1,-1,-1]}}
      mask prompts: edge "Edge Type"; polarity "Output Polarity"; xin "Input X Positions"; yin "Input Y Positions"; xout "Output X Positions"; yout "Output Y Positions"
      mask help: Output is active for one-cycle after each edge of the specified type (i.e. rising, falling or both).
      mask init:
      | edge_detect_init(gcb,edge,polarity);
      settings: AttributesFormatString=|
      | rising edge
      | active high
      mask Help: Output is active for one-cycle after each edge of the specified type (i.e. rising, falling, or both).  Latency is zero.
      mask StyleString: popup(Rising|Falling|Both),popup(Active High|Active Low),edit,edit,edit,edit
      mask Display:
      | plot(xin,0.5+yin{edge}*0.2)
      | plot(xout,0.5+yout{edge}*0.2*(3-2*polarity))
  sync_out : Outport
  dv : Outport  Port=2
  wires:
  bit_slicer/1(zero) -> Mux/2
  bit_slicer/2(b0_0) -> Mux/3
  bit_slicer/3(b1_0) -> Mux/4
  bit_slicer/4(b2_0) -> Mux/5
  bit_slicer/5(b3_0) -> Mux/6
  bit_slicer/6(b4_0) -> Mux/7
  bit_slicer/7(b5_0) -> Mux/8
  bit_slicer/8(b6_0) -> Mux/9
  Counter/1 -> bit_slicer/1(in)
  Register2/1 -> Mux/1
  Mux/1 -> Relational/2
  sync_in/1 -> edge_detect/1(in)
  Constant2/1 -> Relational/1
  edge_detect/1(out) -> Counter/1, Register2/2, Delay/1
  Delay/1 -> sync_out/1
  Relational/1 -> dv/1
  [ds_sel] -> Register2/1

== system fboard_xaui/downsample/dvgen ==
  note: This dvgen block generates a dv signal based on sync_in's rising
      | edge and the value of ds_sel (downsample select), which is taken
      | from a global goto tag.  ds_sel can range from 0 to 7.  The dv
      | signal will be asserted for one cycle every 2^ds_sel cycles starting
      | with the first cycle after sync_out's rising edge.  Note that sync_in
      | may be one or many cycles wide, but it should probably be no
      | wider than 2^ds_sel cycles for typical usage.  sync_out is always
      | one cycle wide (corresponding to the first active cycle of sync_in).
  note: == Example Timing Diagrams ==
      |
      | -------  ds_sel == 0  -------
      | sync_in : .S................
      | sync_out : ....S.............
      | dv : 111111111111111111
      |
      | -------  ds_sel == 1  -------
      | sync_in : .S................
      | sync_out : ....S.............
      | dv : XXXX1.1.1.1.1.1.1.
      |
      | -------  ds_sel == 2  -------
      | sync_in : .SSSS.............
      | sync_out : ....S.............
      | dv : XXXX1...1...1...1.
  note: Only honor new ds_sel value
      | on rising edge of sync_in
  sync_in : Inport  Port=1  LatchInput=off
  Constant2 : xbsIndex_r3/Constant  const=0  equ=P=C  arith_type=Unsigned  n_bits=1  bin_pt=0  opselect=C  inp2=PCIN>>17  opr=+  inp1=P  carry=CIN  iostate=0  explicit_period=on  period=1  dbl_ovrd=off
  Counter : xbsIndex_r3/Counter  cnt_type=Free Running  n_bits=7  bin_pt=0  arith_type=Unsigned  start_count=0  cnt_to=Inf  cnt_by_val=1  operation=Up  explicit_period=off  period=1  load_pin=off  rst=on  en=off  dbl_ovrd=off  show_param=on  use_rpm=on  gen_core=off
      settings: xl_area=[0, 0, 0, 0, 0, 0, 0]
  Delay : xbsIndex_r3/Delay  latency=3  reg_retiming=off  explicit_period=off  period=1  en=off  accept_only_valid=off  init_zero=on  dbl_ovrd=off  show_param=off
      settings: xl_area=[0, 0, 0, 0, 0, 0, 0]
  Mux : xbsIndex_r3/Mux  inputs=8  precision=Full  arith_type="Signed  (2's comp)"  n_bits=8  bin_pt=2  quantization=Truncate  overflow=Wrap  latency=1  explicit_period=off  period=1  en=off  dbl_ovrd=off  show_param=off  mux_type=off  use_rpm=off  gen_core=off
      settings: xl_area=[0, 0, 0, 0, 0, 0, 0]
  Register2 : xbsIndex_r3/Register  init=0  reg_only_valid=off  explicit_period=off  period=1  rst=off  en=on  out_en=off  dbl_ovrd=off  show_param=off
      settings: xl_area=[0, 0, 0, 0, 0, 0, 0]
  Relational : xbsIndex_r3/Relational  mode=a=b  latency=1  explicit_period=off  period=1  en=off  dbl_ovrd=off  show_param=on
      settings: xl_area=[0, 0, 0, 0, 0, 0, 0]
  bit_slicer : Subsystem
  edge_detect : Subsystem  mask(Edge Detector){edge=Rising, polarity=Active High, xin=floor([0.5:0.5:5])*0.08, yin={[-1,-1,1,1,1,1,1,1,1,1],[1,1,-1,-1,-1,-1,-1,-1,-1,-1],[-1,-1,1,1,1,1,-1,-1,-1,-1]}, xout=1-floor([5:-0.5:0.5])*0.08, yout={[-1,-1,1,1,-1,-1,-1,-1,-1,-1],[-1,-1,1,1,-1,-1,-1,-1,-1,-1],[-1,-1,1,1,-1,-1,1,1,-1,-1]}}
      mask prompts: edge "Edge Type"; polarity "Output Polarity"; xin "Input X Positions"; yin "Input Y Positions"; xout "Output X Positions"; yout "Output Y Positions"
      mask help: Output is active for one-cycle after each edge of the specified type (i.e. rising, falling or both).
      mask init:
      | edge_detect_init(gcb,edge,polarity);
      settings: AttributesFormatString=|
      | rising edge
      | active high
      mask Help: Output is active for one-cycle after each edge of the specified type (i.e. rising, falling, or both).  Latency is zero.
      mask StyleString: popup(Rising|Falling|Both),popup(Active High|Active Low),edit,edit,edit,edit
      mask Display:
      | plot(xin,0.5+yin{edge}*0.2)
      | plot(xout,0.5+yout{edge}*0.2*(3-2*polarity))
  sync_out : Outport
  dv : Outport  Port=2
  wires:
  bit_slicer/1(zero) -> Mux/2
  bit_slicer/2(b0_0) -> Mux/3
  bit_slicer/3(b1_0) -> Mux/4
  bit_slicer/4(b2_0) -> Mux/5
  bit_slicer/5(b3_0) -> Mux/6
  bit_slicer/6(b4_0) -> Mux/7
  bit_slicer/7(b5_0) -> Mux/8
  bit_slicer/8(b6_0) -> Mux/9
  Counter/1 -> bit_slicer/1(in)
  Register2/1 -> Mux/1
  Mux/1 -> Relational/2
  sync_in/1 -> edge_detect/1(in)
  Constant2/1 -> Relational/1
  edge_detect/1(out) -> Counter/1, Register2/2, Delay/1
  Delay/1 -> sync_out/1
  Relational/1 -> dv/1
  [ds_sel] -> Register2/1

== system fboard_xaui/pfb8/b64x1_b16x4_bot ==
  din : Inport  Port=1  LatchInput=off
  Slice0 : xbsIndex_r3/Slice  mode=Lower Bit Location + Width  nbits=16  bit1=0  base1=LSB of Input  bit0=0  base0=LSB of Input  boolean_output=off  explicit_period=off  period=1  dbl_ovrd=off
  Slice1 : xbsIndex_r3/Slice  mode=Lower Bit Location + Width  nbits=16  bit1=0  base1=LSB of Input  bit0=16  base0=LSB of Input  boolean_output=off  explicit_period=off  period=1  dbl_ovrd=off
  Slice2 : xbsIndex_r3/Slice  mode=Lower Bit Location + Width  nbits=16  bit1=0  base1=LSB of Input  bit0=32  base0=LSB of Input  boolean_output=off  explicit_period=off  period=1  dbl_ovrd=off
  Slice3 : xbsIndex_r3/Slice  mode=Lower Bit Location + Width  nbits=16  bit1=0  base1=LSB of Input  bit0=48  base0=LSB of Input  boolean_output=off  explicit_period=off  period=1  dbl_ovrd=off
  dout0 : Outport
  dout1 : Outport  Port=2
  dout2 : Outport  Port=3
  dout3 : Outport  Port=4
  wires:
  Slice0/1 -> dout3/1
  Slice1/1 -> dout2/1
  Slice2/1 -> dout1/1
  Slice3/1 -> dout0/1
  din/1 -> Slice1/1, Slice0/1, Slice2/1, Slice3/1

== system fboard_xaui/pfb8/b64x1_b16x4_top ==
  din : Inport  Port=1  LatchInput=off
  Slice0 : xbsIndex_r3/Slice  mode=Lower Bit Location + Width  nbits=16  bit1=0  base1=LSB of Input  bit0=0  base0=LSB of Input  boolean_output=off  explicit_period=off  period=1  dbl_ovrd=off
  Slice1 : xbsIndex_r3/Slice  mode=Lower Bit Location + Width  nbits=16  bit1=0  base1=LSB of Input  bit0=16  base0=LSB of Input  boolean_output=off  explicit_period=off  period=1  dbl_ovrd=off
  Slice2 : xbsIndex_r3/Slice  mode=Lower Bit Location + Width  nbits=16  bit1=0  base1=LSB of Input  bit0=32  base0=LSB of Input  boolean_output=off  explicit_period=off  period=1  dbl_ovrd=off
  Slice3 : xbsIndex_r3/Slice  mode=Lower Bit Location + Width  nbits=16  bit1=0  base1=LSB of Input  bit0=48  base0=LSB of Input  boolean_output=off  explicit_period=off  period=1  dbl_ovrd=off
  dout0 : Outport
  dout1 : Outport  Port=2
  dout2 : Outport  Port=3
  dout3 : Outport  Port=4
  wires:
  din/1 -> Slice3/1, Slice2/1, Slice0/1, Slice1/1
  Slice3/1 -> dout0/1
  Slice2/1 -> dout1/1
  Slice1/1 -> dout2/1
  Slice0/1 -> dout3/1

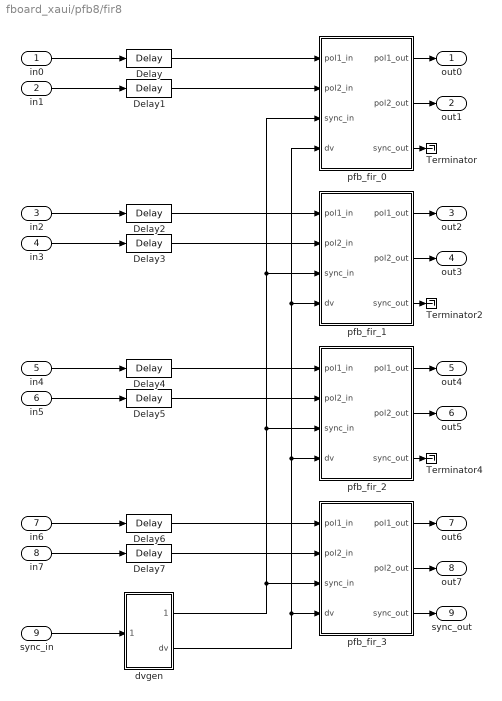
== system fboard_xaui/pfb8/fir8 ==
  in0 : Inport  Port=1  LatchInput=off
  in1 : Inport  Port=2  LatchInput=off
  in2 : Inport  Port=3  LatchInput=off
  in3 : Inport  Port=4  LatchInput=off
  in4 : Inport  Port=5  LatchInput=off
  in5 : Inport  Port=6  LatchInput=off
  in6 : Inport  Port=7  LatchInput=off
  in7 : Inport  Port=8  LatchInput=off
  sync_in : Inport  Port=9  LatchInput=off
  Delay{,1..7} (8 alike) : xbsIndex_r3/Delay  latency=3  reg_retiming=off  explicit_period=off  period=1  en=off  accept_only_valid=off  init_zero=on  dbl_ovrd=off  show_param=off
      settings: xl_area=[0, 0, 0, 0, 0, 0, 0]
  Terminator : Terminator
  Terminator2 : Terminator
  Terminator4 : Terminator
  dvgen : Subsystem
      settings: AttributesFormatString=Latency=3
  pfb_fir_0 : Subsystem
  pfb_fir_1 : Subsystem
  pfb_fir_2 : Subsystem
  pfb_fir_3 : Subsystem
  out0 : Outport
  out1 : Outport  Port=2
  out2 : Outport  Port=3
  out3 : Outport  Port=4
  out4 : Outport  Port=5
  out5 : Outport  Port=6
  out6 : Outport  Port=7
  out7 : Outport  Port=8
  sync_out : Outport  Port=9
  wires:
  in0/1 -> Delay/1
  pfb_fir_0/1(pol1_out) -> out0/1
  in1/1 -> Delay1/1
  pfb_fir_0/2(pol2_out) -> out1/1
  in2/1 -> Delay2/1
  pfb_fir_1/1(pol1_out) -> out2/1
  in3/1 -> Delay3/1
  pfb_fir_1/2(pol2_out) -> out3/1
  in4/1 -> Delay4/1
  pfb_fir_2/1(pol1_out) -> out4/1
  in5/1 -> Delay5/1
  pfb_fir_2/2(pol2_out) -> out5/1
  dvgen/1(sync_out) -> pfb_fir_0/3(sync_in), pfb_fir_1/3(sync_in), pfb_fir_2/3(sync_in), pfb_fir_3/3(sync_in)
  pfb_fir_3/3(sync_out) -> sync_out/1
  in6/1 -> Delay6/1
  pfb_fir_3/1(pol1_out) -> out6/1
  pfb_fir_3/2(pol2_out) -> out7/1
  in7/1 -> Delay7/1
  pfb_fir_0/3(sync_out) -> Terminator/1
  pfb_fir_1/3(sync_out) -> Terminator2/1
  pfb_fir_2/3(sync_out) -> Terminator4/1
  dvgen/2(dv) -> pfb_fir_0/4(dv), pfb_fir_1/4(dv), pfb_fir_2/4(dv), pfb_fir_3/4(dv)
  sync_in/1 -> dvgen/1(sync_in)
  Delay/1 -> pfb_fir_0/1(pol1_in)
  Delay1/1 -> pfb_fir_0/2(pol2_in)
  Delay2/1 -> pfb_fir_1/1(pol1_in)
  Delay3/1 -> pfb_fir_1/2(pol2_in)
  Delay4/1 -> pfb_fir_2/1(pol1_in)
  Delay5/1 -> pfb_fir_2/2(pol2_in)
  Delay6/1 -> pfb_fir_3/1(pol1_in)
  Delay7/1 -> pfb_fir_3/2(pol2_in)

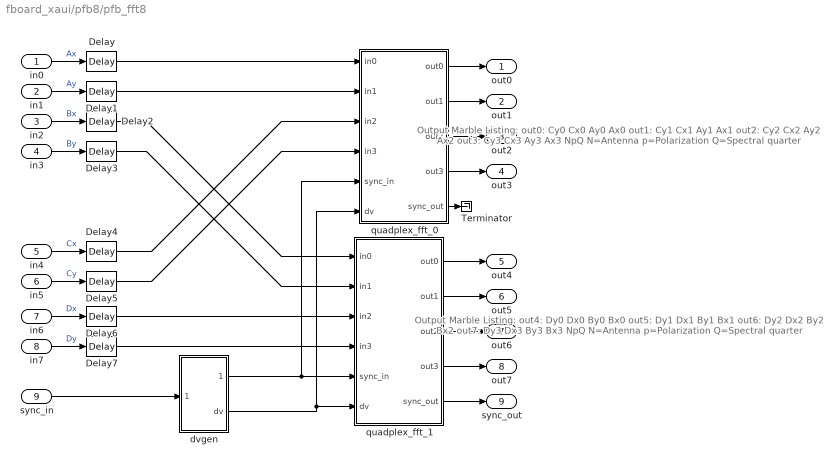
== system fboard_xaui/pfb8/pfb_fft8 ==
  note: Output Marble Listing:
      |
      | out0: Cy0 Cx0 Ay0 Ax0
      | out1: Cy1 Cx1 Ay1 Ax1
      | out2: Cy2 Cx2 Ay2 Ax2
      | out3: Cy3 Cx3 Ay3 Ax3
      |
      | NpQ
      | N=Antenna
      | p=Polarization
      | Q=Spectral quarter
  note: Output Marble Listing:
      |
      | out4: Dy0 Dx0 By0 Bx0
      | out5: Dy1 Dx1 By1 Bx1
      | out6: Dy2 Dx2 By2 Bx2
      | out7: Dy3 Dx3 By3 Bx3
      |
      | NpQ
      | N=Antenna
      | p=Polarization
      | Q=Spectral quarter
  in0 : Inport  Port=1  LatchInput=off
  in1 : Inport  Port=2  LatchInput=off
  in2 : Inport  Port=3  LatchInput=off
  in3 : Inport  Port=4  LatchInput=off
  in4 : Inport  Port=5  LatchInput=off
  in5 : Inport  Port=6  LatchInput=off
  in6 : Inport  Port=7  LatchInput=off
  in7 : Inport  Port=8  LatchInput=off
  sync_in : Inport  Port=9  LatchInput=off
  Delay{,1..7} (8 alike) : xbsIndex_r3/Delay  latency=3  reg_retiming=off  explicit_period=off  period=1  en=off  accept_only_valid=off  init_zero=on  dbl_ovrd=off  show_param=off
      settings: xl_area=[0, 0, 0, 0, 0, 0, 0]
  Terminator : Terminator
  dvgen : Subsystem
      settings: AttributesFormatString=Latency=3
  quadplex_fft_0 : Subsystem
  quadplex_fft_1 : Subsystem
  out0 : Outport
  out1 : Outport  Port=2
  out2 : Outport  Port=3
  out3 : Outport  Port=4
  out4 : Outport  Port=5
  out5 : Outport  Port=6
  out6 : Outport  Port=7
  out7 : Outport  Port=8
  sync_out : Outport  Port=9
  wires:
  in0/1 -> Delay/1  "Ax"
  quadplex_fft_0/1(out0) -> out0/1
  in1/1 -> Delay1/1  "Ay"
  quadplex_fft_0/2(out1) -> out1/1
  quadplex_fft_0/3(out2) -> out2/1
  quadplex_fft_0/4(out3) -> out3/1
  quadplex_fft_1/1(out0) -> out4/1
  quadplex_fft_1/2(out1) -> out5/1
  in6/1 -> Delay6/1  "Dx"
  quadplex_fft_1/3(out2) -> out6/1
  in7/1 -> Delay7/1  "Dy"
  quadplex_fft_1/4(out3) -> out7/1
  dvgen/1(sync_out) -> quadplex_fft_0/5(sync_in), quadplex_fft_1/5(sync_in)
  quadplex_fft_1/5(sync_out) -> sync_out/1
  quadplex_fft_0/5(sync_out) -> Terminator/1
  in2/1 -> Delay2/1  "Bx"
  in3/1 -> Delay3/1  "By"
  in4/1 -> Delay4/1  "Cx"
  in5/1 -> Delay5/1  "Cy"
  Delay/1 -> quadplex_fft_0/1(in0)
  Delay1/1 -> quadplex_fft_0/2(in1)
  Delay2/1 -> quadplex_fft_1/1(in0)
  Delay3/1 -> quadplex_fft_1/2(in1)
  Delay4/1 -> quadplex_fft_0/3(in2)
  Delay5/1 -> quadplex_fft_0/4(in3)
  Delay6/1 -> quadplex_fft_1/3(in2)
  Delay7/1 -> quadplex_fft_1/4(in3)
  sync_in/1 -> dvgen/1(sync_in)
  dvgen/2(dv) -> quadplex_fft_0/6(dv), quadplex_fft_1/6(dv)

== system fboard_xaui/xaui/llc ==
  in : Inport  Port=1  LatchInput=off
  Counter : xbsIndex_r3/Counter  cnt_type=Free Running  n_bits=16  bin_pt=0  arith_type="Signed  (2's comp)"  start_count=0  cnt_to=Inf  cnt_by_val=1  operation=Up  explicit_period=off  period=1  load_pin=on  rst=off  en=on  dbl_ovrd=off  show_param=off  use_rpm=on  gen_core=off
      settings: xl_area=[0, 0, 0, 0, 0, 0, 0]
  Logical : xbsIndex_r3/Logical  logical_function=OR  inputs=2  precision=Full  arith_type=Unsigned  n_bits=8  bin_pt=2  align_bp=on  latency=0  explicit_period=off  period=1  en=off  dbl_ovrd=off  show_param=off
      settings: xl_area=[0, 0, 0, 0, 0, 0, 0]
  Negate : xbsIndex_r3/Negate  precision=Full  arith_type="Signed  (2's comp)"  n_bits=16  bin_pt=0  quantization=Truncate  overflow=Wrap  latency=1  explicit_period=off  period=1  en=off  dbl_ovrd=off  use_core=on  show_param=off  use_rpm=on  gen_core=off
      settings: xl_area=[0, 0, 0, 0, 0, 0, 0]
  b14_b0 : xbsIndex_r3/Slice  mode=Lower Bit Location + Width  nbits=15  bit1=0  base1=MSB of Input  bit0=0  base0=LSB of Input  boolean_output=off  explicit_period=off  period=1  dbl_ovrd=off
  falling_edge : Subsystem
  msb : xbsIndex_r3/Slice  mode=Upper Bit Location + Width  nbits=1  bit1=0  base1=MSB of Input  bit0=0  base0=LSB of Input  boolean_output=on  explicit_period=off  period=1  dbl_ovrd=off
  rising_edge : Subsystem
  out : Outport
  wires:
  rising_edge/1(out) -> Counter/1, Logical/1
  in/1 -> rising_edge/1(in)
  Counter/1 -> msb/1
  msb/1 -> Logical/2
  b14_b0/1 -> Negate/1
  Negate/1 -> Counter/2
  [reg1] -> b14_b0/1
  falling_edge/1(out) -> out/1
  Logical/1 -> Counter/3, falling_edge/1(in)
